simulink model "faragasso_dynamics"  (R2014b)
settings: Solver=ode45  StartTime=0.0  StopTime=1000  RelTol=1e-3
values from neighbouring files (symbols this model uses):
  k1 = 0.001    [faragasso_params.m]
  k2 = 0.0034    [faragasso_params.m]
  k3 = 0.00787    [faragasso_params.m]
  L1 = -0.1    [faragasso_params.m]
  L2 = -0.1    [faragasso_params.m]
  theta0 = 0    [faragasso_params.m]
  v = 5    [faragasso_params.m]
  x0 = 0    [faragasso_params.m]
  xm0 = 0.1    [faragasso_params.m]
  xv0 = .1    (= 0.1)    [faragasso_params.m]
  y0 = 0    [faragasso_params.m]
settings Model: Creator=root  LastModifiedBy=root

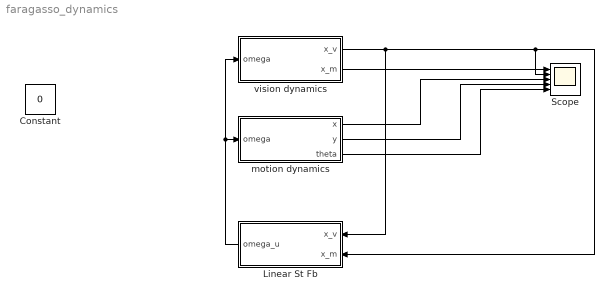
== system faragasso_dynamics ==
  Constant : Constant  Value=0
  Linear St Fb : Subsystem
  Scope : Scope  NumInputPorts=5
      settings: YMin=-5~-5~-5~-5~-5  YMax=5~5~5~5~5
  motion dynamics : Subsystem
  vision dynamics : Subsystem
  wires:
  vision dynamics/2(x_m) -> Scope/2
  vision dynamics/1(x_v) -> Linear St Fb/1(x_v), Linear St Fb/2(x_m), Scope/1
  motion dynamics/1(x) -> Scope/3
  motion dynamics/2(y) -> Scope/4
  motion dynamics/3(theta) -> Scope/5
  Linear St Fb/1(omega_u) -> motion dynamics/1(omega), vision dynamics/1(omega)

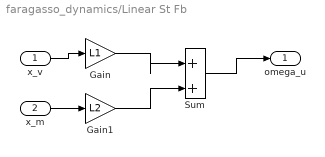
== system faragasso_dynamics/Linear St Fb ==
  x_v : Inport
  x_m : Inport  Port=2
  Gain : Gain  Gain=L1
  Gain1 : Gain  Gain=L2
  Sum : Sum  Inputs=|++
  omega_u : Outport
  wires:
  Sum/1 -> omega_u/1
  x_v/1 -> Gain/1
  x_m/1 -> Gain1/1
  Gain/1 -> Sum/1
  Gain1/1 -> Sum/2

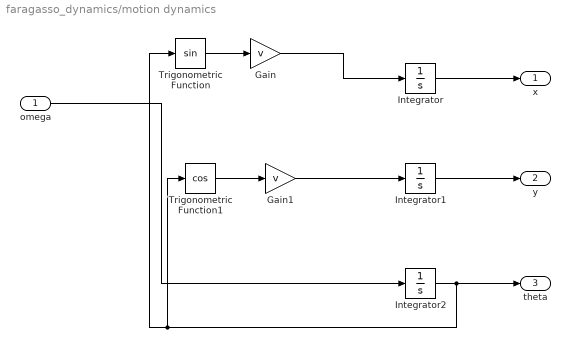
== system faragasso_dynamics/motion dynamics ==
  omega : Inport
  Gain : Gain  Gain=v
  Gain1 : Gain  Gain=v
  Integrator : Integrator  InitialCondition=x0
  Integrator1 : Integrator  InitialCondition=y0
  Integrator2 : Integrator  InitialCondition=theta0
  Trigonometric Function : Trigonometry
  Trigonometric Function1 : Trigonometry  Operator=cos
  x : Outport
  y : Outport  Port=2
  theta : Outport  Port=3
  wires:
  Integrator2/1 -> theta/1, Trigonometric Function/1, Trigonometric Function1/1
  Trigonometric Function/1 -> Gain/1
  Gain/1 -> Integrator/1
  Integrator/1 -> x/1
  Trigonometric Function1/1 -> Gain1/1
  Gain1/1 -> Integrator1/1
  Integrator1/1 -> y/1
  omega/1 -> Integrator2/1

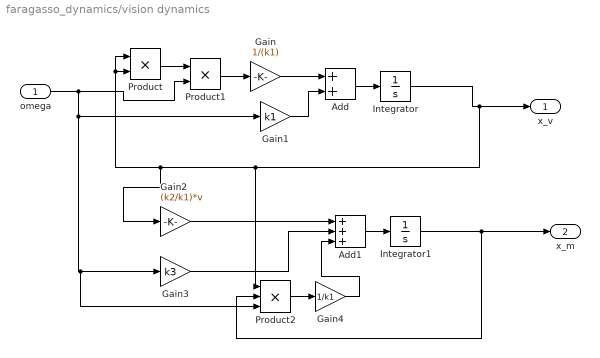
== system faragasso_dynamics/vision dynamics ==
  omega : Inport
  Add : Sum
  Add1 : Sum  Inputs=+++
  Gain : Gain  Gain=1/(k1)
  Gain1 : Gain  Gain=k1
  Gain2 : Gain  Gain=(k2/k1)*v
  Gain3 : Gain  Gain=k3
  Gain4 : Gain  Gain=1/k1
  Integrator : Integrator  InitialCondition=xv0
  Integrator1 : Integrator  InitialCondition=xm0
  Product : Product
  Product1 : Product
  Product2 : Product  Inputs=3
  x_v : Outport
  x_m : Outport  Port=2
  wires:
  Product/1 -> Product1/1
  omega/1 -> Product2/3, Gain3/1, Gain1/1, Product1/2
  Product1/1 -> Gain/1
  Gain/1 -> Add/1
  Gain1/1 -> Add/2
  Integrator1/1 -> Product2/2, x_m/1
  Integrator/1 -> Product2/1, Gain2/1, Product/1, Product/2, x_v/1
  Product2/1 -> Gain4/1
  Add1/1 -> Integrator1/1
  Gain4/1 -> Add1/3
  Gain2/1 -> Add1/1
  Gain3/1 -> Add1/2
  Add/1 -> Integrator/1
